simulink model "ManeuverPlanning"  (R2020b)
settings: Solver=FixedStepAuto  StartTime=0.0  StopTime=15  FixedStep=Ts/2  RelTol=1e-3
values from neighbouring files (symbols this model uses):
  Ts = 0.01    [prepare_simulation.m]
undefined symbols (not defined in the file or in its folder): constraints, dimensionsEgo, dimensionsLead, ego, laneWidth, lateral, other, road, roadTrajectory, uncertainty, v_max, v_min, wheelBaseEgo, wheelBaseLead, xEgo_0, yawEgo_0, yEgo_0
libraries: sim3dautolib x3, mpcadaslib x2, vrlib x2, simulink x2, robotalgslib x1, drivingvehiclecontroller x1, pid_lib x1, sim3dlib x1, robotmobilelib x1
(part 2 of 2)

== matlab function ManeuverPlanning/Unused Blocks/MATLAB Function ==
  data: poseVehicle1 input; egoTrajectory input; nextWpsPurePursuit input; poseVehicle2 input; dimensionsVehicle1 parameter; wheelBaseVehicle1 parameter; dimensionsVehicle2 parameter; wheelBaseVehicle2 parameter; LaneWidth parameter; roadTrajectory parameter
function plotVehicles(poseVehicle1, egoTrajectory, nextWpsPurePursuit, poseVehicle2, dimensionsVehicle1, wheelBaseVehicle1, dimensionsVehicle2, wheelBaseVehicle2, LaneWidth, roadTrajectory)
% Plot vehicles and road and trajectory followed by the ego vehicle
    
    % Clear previous Vehicle
    cla;
    
    % Vehicle 1
    [plotVehicle1, plotVehicleLocation1] = plotVehicle(poseVehicle1, wheelBaseVehicle1, dimensionsVehicle1, 'g', 'o');
    % Traces
    
    
    % Vehicle 2
    [plotVehicle2, plotVehicleLocation2] = plotVehicle(poseVehicle2, wheelBaseVehicle2, dimensionsVehicle2, 'r', 'o');
    
    % Road 
    plotRoad(roadTrajectory, LaneWidth);
    
    % Trajectory
    plotTrajectory = plot(egoTrajectory(:, 1), egoTrajectory(:, 2), 'Color', 'green');
    plotWPs = plot(nextWpsPurePursuit(:, 1), nextWpsPurePursuit(:, 2), '-*');

    % Adjust Axis
    x2 = poseVehicle2(1);
    y2 = poseVehicle2(2);
    axis([x2-40 x2+40 y2-20 y2+20]); % Camera following V2 as ego vehicle
end

function [plotVehicle, plotVehicleLocation] = plotVehicle(poseRearAxle, wheelBase, dim, color, originRepresentation)
% Plot vehicle

    centerPoint = getVehicleCenterPoint(poseRearAxle, wheelBase);

    [corners_x, corners_y, ~] = createRectangleVehicle(centerPoint, poseRearAxle(3), dim);
    
    plotVehicle = plot(corners_x, corners_y, color); % Vehicle rectangle
    plotVehicleLocation = plot(poseRearAxle(1), poseRearAxle(2), originRepresentation, 'Color', 'black'); % Vehicle location
end

function plotRoad(roadTrajectory, laneWidth)
% Plot road

    route = roadTrajectory([1, 2],[1, 3]).*[1, -1; 1, -1];
    radian = roadTrajectory(3, 1);
    startPoint = route(1, :);
    endPoint = route(2, :);
    
    lineOffset = -laneWidth/2; % Offset for each line: Start with lower line

    if radian == 0 % Straight road
        route_Vector = endPoint - startPoint;
        routeUnitVector = route_Vector/norm(route_Vector);% unit vector of the route_vector
        routeNormalUnitVector = [-routeUnitVector(2), routeUnitVector(1)]; % Route normal unit vector

        for lineNr = 1:3 % For lower, middle and upper line
            startLine = startPoint + lineOffset*routeNormalUnitVector;
            endLine = endPoint + lineOffset*routeNormalUnitVector;
            
            lineOffset = plotRoadLine([startLine(1), endLine(1)], [startLine(2), endLine(2)], lineNr, lineOffset, laneWidth);
        end
    else % Curved road
        rotationCenter = roadTrajectory(3, [2, 3]).*[1, -1]; 
        startPointVector = startPoint - rotationCenter;
        routeRadius = norm(startPointVector); 
        startPointVectorAng = atan2(startPointVector(2),startPointVector(1)); 

        angles = startPointVectorAng:radian/(0.2*routeRadius*radian/pi):startPointVectorAng+radian; % Discretise angles from start to end point

        for lineNr = 1:3 % For lower, middle and upper line
            x_arc = rotationCenter(1) + (routeRadius-lineOffset)*cos(angles);
            y_arc = rotationCenter(2) + (routeRadius-lineOffset)*sin(angles);
            
            lineOffset = plotRoadLine(x_arc, y_arc, lineNr, lineOffset, laneWidth);
        end  
    end
end

function lineOffset = plotRoadLine(x_line, y_line, lineNr, lineOffset, laneWidth)
% Plot current road line, return offset for next line

    lineRepresentation = '-';
    if lineNr == 2 % Dashed for middle line
        lineRepresentation = '--';
    end

    plot(x_line, y_line, lineRepresentation, 'Color', 'blue');
    
    lineOffset = lineOffset + laneWidth; % Next line
end

== matlab function ManeuverPlanning/Ego Vehicle/Lateral Error - PID/MATLAB Function ==
  data: s output; x input; y input; d output; currentTrajectory parameter
function [s, d] = Cartesian2FrenetBlock(x, y, currentTrajectory)
% Simulink block for Frenet2Cartesian

    [s, d] = Cartesian2Frenet(currentTrajectory, [x, y]);
end

== matlab function ManeuverPlanning/Ego Vehicle/Vehicle Following Mode/MATLAB Function ==
  data: delta_s_lead output; ids_surroundingVehicles input; distances_surroundingVehicles input; vLead output; speedsOtherVehicles input
function [delta_s_lead, vLead] = getLeadingVehicleInformation(ids_surroundingVehicles, distances_surroundingVehicles, speedsOtherVehicles)
% Get speed of and distance to leading vehicle
    
    % PID controller needs some values even if there is no detection:
    delta_s_lead = 9999; % Singulatity for distance = inf
    vLead = 0;
    
    id_leadingVehicle = ids_surroundingVehicles(1);
    
    if id_leadingVehicle ~= -1 % Vehicle detected
        delta_s_lead = distances_surroundingVehicles(1);
        vLead = speedsOtherVehicles(id_leadingVehicle);
    end
end
